simulink model "sim3_2"  (R2019a)
settings: Solver=VariableStepAuto  StartTime=0.0  StopTime=10.0  RelTol=1e-3
values from neighbouring files (symbols this model uses):
  denG = [1 3.74 0]    [matlab3_2.m]
  Kd = (2 * ksi * wn + p - denG(2))/numG(1)    [matlab3_2.m]
  Ki = (p * wn^2)/numG(1)    [matlab3_2.m]
  Kp = (2 * p * ksi * wn + wn^2 - denG(3))/numG(1)    [matlab3_2.m]
  numG = [2.05]    [matlab3_2.m]
settings Model: Creator=User  LastModifiedBy=User

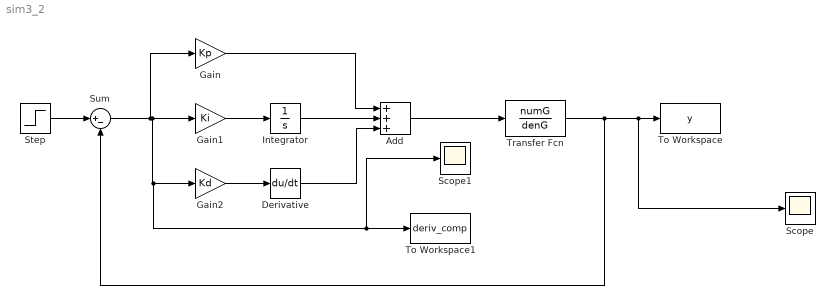
== system sim3_2 ==
  Add : Sum  Inputs=+++
  Derivative : Derivative
  Gain : Gain  Gain=Kp
  Gain1 : Gain  Gain=Ki
  Gain2 : Gain  Gain=Kd
  Integrator : Integrator
  Scope : Scope
  Scope1 : Scope
  Step : Step  SampleTime=0
  Sum : Sum  Inputs=|+-
  To Workspace : ToWorkspace  VariableName=y  SaveFormat=Structure With Time  SampleTime=-1
  To Workspace1 : ToWorkspace  VariableName=deriv_comp  SaveFormat=Structure With Time  SampleTime=-1
  Transfer Fcn : TransferFcn  Numerator=numG  Denominator=denG
  wires:
  Sum/1 -> Gain/1, Scope1/1, To Workspace1/1, Gain2/1, Gain1/1
  Gain2/1 -> Derivative/1
  Gain1/1 -> Integrator/1
  Integrator/1 -> Add/2
  Gain/1 -> Add/1
  Derivative/1 -> Add/3
  Transfer Fcn/1 -> Sum/2, Scope/1, To Workspace/1
  Step/1 -> Sum/1
  Add/1 -> Transfer Fcn/1
